simulink model "bicyclemodel22"  (R2015b)
settings: Solver=FixedStepAuto  StartTime=0.0  StopTime=1  FixedStep=0.001  RelTol=1e-3
libraries: simulink x3
settings Model: Creator=ADMIN  LastModifiedBy=ADMIN

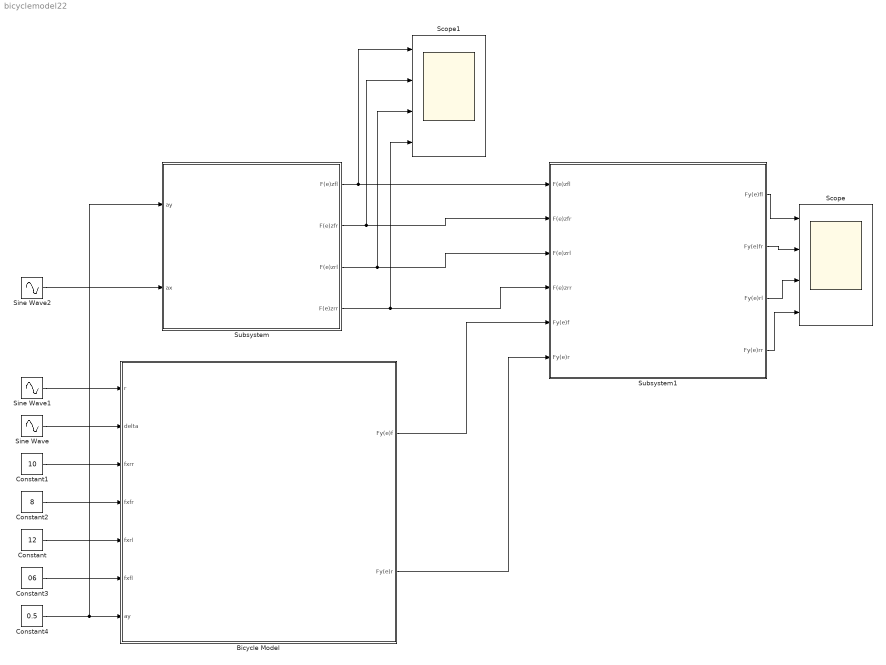
== system bicyclemodel22 ==
  Bicycle Model : Subsystem
  Constant : Constant  Value=12
  Constant1 : Constant  Value=10
  Constant2 : Constant  Value=8
  Constant3 : Constant  Value=06
  Constant4 : Constant  Value=0.5
  Scope : Scope  NumInputPorts=4
  Scope1 : Scope  NumInputPorts=4
  Sine Wave : Sin  Frequency=2
  Sine Wave1 : Sin  Frequency=4
  Sine Wave2 : Sin  Frequency=5
  Subsystem : Subsystem
  Subsystem1 : Subsystem
  wires:
  Subsystem/1(F(e)zfl) -> Scope1/1, Subsystem1/1(F(e)zfl)
  Subsystem/2(F(e)zfr) -> Scope1/2, Subsystem1/2(F(e)zfr)
  Subsystem/3(F(e)zrl) -> Scope1/3, Subsystem1/3(F(e)zrl)
  Subsystem/4(F(e)zrr) -> Scope1/4, Subsystem1/4(F(e)zrr)
  Bicycle Model/1(Fy(e)f) -> Subsystem1/5(Fy(e)f)
  Bicycle Model/2(Fy(e)r) -> Subsystem1/6(Fy(e)r)
  Constant/1 -> Bicycle Model/5(fxrl)
  Sine Wave/1 -> Bicycle Model/2(delta)
  Constant3/1 -> Bicycle Model/6(fxfl)
  Constant2/1 -> Bicycle Model/4(fxfr)
  Constant1/1 -> Bicycle Model/3(fxrr)
  Constant4/1 -> Subsystem/1(ay), Bicycle Model/7(ay)
  Sine Wave1/1 -> Bicycle Model/1(r)
  Subsystem1/1(Fy(e)fl) -> Scope/1
  Sine Wave2/1 -> Subsystem/2(ax)
  Subsystem1/2(Fy(e)fr) -> Scope/2
  Subsystem1/3(Fy(e)rl) -> Scope/3
  Subsystem1/4(Fy(e)rr) -> Scope/4

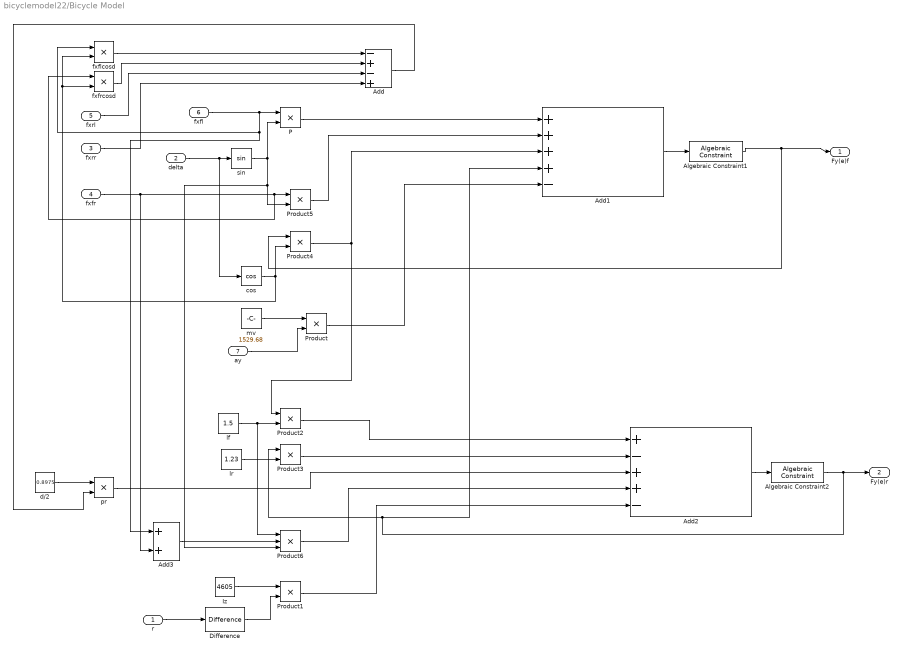
== system bicyclemodel22/Bicycle Model ==
  r : Inport
  delta : Inport  Port=2
  fxrr : Inport  Port=3
  fxfr : Inport  Port=4
  fxrl : Inport  Port=5
  fxfl : Inport  Port=6
  ay : Inport  Port=7
  Add : Sum  Inputs=-+-+
  Add1 : Sum  Inputs=++++-
  Add2 : Sum  Inputs=+-++-
  Add3 : Sum
  Algebraic Constraint1 : simulink/Math Operations/Algebraic Constraint  z0=0
  Algebraic Constraint2 : simulink/Math Operations/Algebraic Constraint  z0=0
  Difference : simulink/Discrete/Difference  ICPrevInput=0.0  InputProcessing=Inherited  OutMin=[]  OutMax=[]  OutDataType=fixdt(1, 16)  OutScaling=2^-10  DoSatur=off
  Iz : Constant  Value=4605
  P : Product
  Product{,1..5} (6 alike) : Product
  Product6 : Product  Inputs=3
  cos : Trigonometry  Operator=cos
  d/2 : Constant  Value=0.8975
  fxflcosd : Product
  fxfrcosd : Product
  lf : Constant  Value=1.5
  lr : Constant  Value=1.23
  mv : Constant  Value=1529.68
  pr : Product
  sin : Trigonometry
  Fy(e)f : Outport
  Fy(e)r : Outport  Port=2
  wires:
  fxfl/1 -> Add3/1, fxflcosd/1, P/1
  fxflcosd/1 -> Add/1
  Add3/1 -> Product6/2
  Add/1 -> pr/2
  Product6/1 -> Add2/4
  fxrr/1 -> Add/4
  fxrl/1 -> Add/3
  Product1/1 -> Add2/5
  fxfrcosd/1 -> Add/2
  r/1 -> Difference/1
  lr/1 -> Product3/2
  lf/1 -> Product6/1, Product2/2
  Product3/1 -> Add2/2
  Product2/1 -> Add2/1
  Iz/1 -> Product1/1
  Algebraic Constraint1/1 -> Product4/1, Fy(e)f/1
  Algebraic Constraint2/1 -> Product3/1, Add1/4, Fy(e)r/1
  mv/1 -> Product/1
  ay/1 -> Product/2
  P/1 -> Add1/1
  delta/1 -> cos/1, sin/1
  Add1/1 -> Algebraic Constraint1/1
  Add2/1 -> Algebraic Constraint2/1
  fxfr/1 -> fxfrcosd/1, Product5/1, Add3/2
  sin/1 -> Product5/2, Product6/3, P/2
  Product5/1 -> Add1/2
  Product4/1 -> Product2/1, Add1/3
  cos/1 -> fxfrcosd/2, fxflcosd/2, Product4/2
  Product/1 -> Add1/5
  d/2/1 -> pr/1
  pr/1 -> Add2/3
  Difference/1 -> Product1/2

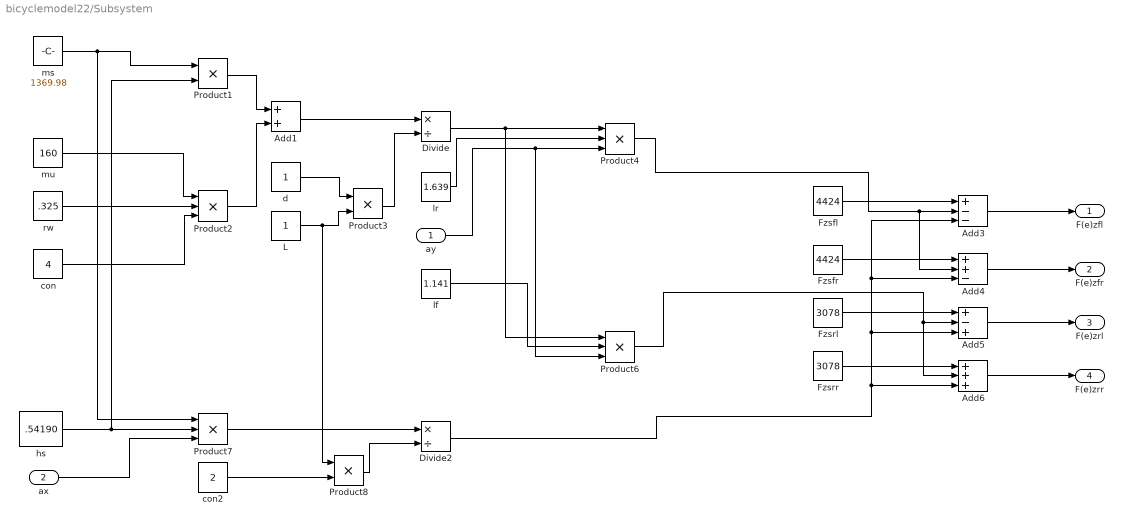
== system bicyclemodel22/Subsystem ==
  ay : Inport
  ax : Inport  Port=2
  Add1 : Sum
  Add3 : Sum  Inputs=+--
  Add4 : Sum  Inputs=++-
  Add5 : Sum  Inputs=+-+
  Add6 : Sum  Inputs=+++
  Divide : Product  Inputs=*/
  Divide2 : Product  Inputs=*/
  Fzsfl : Constant  Value=4424
  Fzsfr : Constant  Value=4424
  Fzsrl : Constant  Value=3078
  Fzsrr : Constant  Value=3078
  L : Constant
  Product1 : Product
  Product{2,4,6..7} (4 alike) : Product  Inputs=3
  Product3 : Product
  Product8 : Product
  con : Constant  Value=4
  con2 : Constant  Value=2
  d : Constant
  hs : Constant  Value=.54190
  lf : Constant  Value=1.141
  lr : Constant  Value=1.639
  ms : Constant  Value=1369.98
  mu : Constant  Value=160
  rw : Constant  Value=.325
  F(e)zfl : Outport
  F(e)zfr : Outport  Port=2
  F(e)zrl : Outport  Port=3
  F(e)zrr : Outport  Port=4
  wires:
  lr/1 -> Product4/2
  ms/1 -> Product7/1, Product1/1
  Divide/1 -> Product6/1, Product4/1
  hs/1 -> Product1/2, Product7/2
  Product3/1 -> Divide/2
  Add1/1 -> Divide/1
  Product1/1 -> Add1/1
  rw/1 -> Product2/2
  Product2/1 -> Add1/2
  mu/1 -> Product2/1
  L/1 -> Product8/1, Product3/2
  d/1 -> Product3/1
  con/1 -> Product2/3
  Product4/1 -> Add4/2, Add3/2
  Product6/1 -> Add6/2, Add5/2
  con2/1 -> Product8/2
  Add6/1 -> F(e)zrr/1
  ax/1 -> Product7/3
  Product7/1 -> Divide2/1
  Fzsrl/1 -> Add5/1
  lf/1 -> Product6/2
  Fzsfl/1 -> Add3/1
  ay/1 -> Product6/3, Product4/3
  Product8/1 -> Divide2/2
  Fzsrr/1 -> Add6/1
  Divide2/1 -> Add6/3, Add5/3, Add4/3, Add3/3
  Add5/1 -> F(e)zrl/1
  Add3/1 -> F(e)zfl/1
  Add4/1 -> F(e)zfr/1
  Fzsfr/1 -> Add4/1

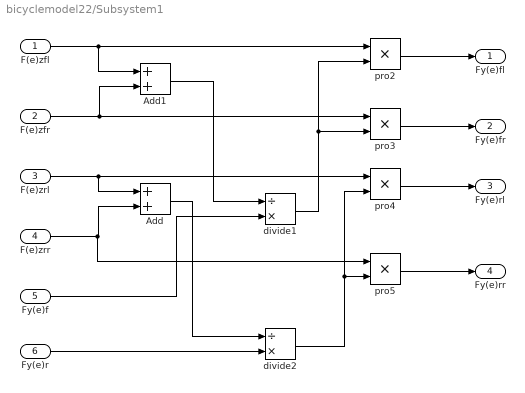
== system bicyclemodel22/Subsystem1 ==
  F(e)zfl : Inport
  F(e)zfr : Inport  Port=2
  F(e)zrl : Inport  Port=3
  F(e)zrr : Inport  Port=4
  Fy(e)f : Inport  Port=5
  Fy(e)r : Inport  Port=6
  Add : Sum
  Add1 : Sum
  divide1 : Product  Inputs=/*
  divide2 : Product  Inputs=/*
  pro{2..5} (4 alike) : Product  Inputs=**
  Fy(e)fl : Outport
  Fy(e)fr : Outport  Port=2
  Fy(e)rl : Outport  Port=3
  Fy(e)rr : Outport  Port=4
  wires:
  Add/1 -> divide2/1
  Fy(e)r/1 -> divide2/2
  F(e)zrl/1 -> pro4/1, Add/1
  divide1/1 -> pro3/2, pro2/2
  pro4/1 -> Fy(e)rl/1
  pro2/1 -> Fy(e)fl/1
  pro3/1 -> Fy(e)fr/1
  Fy(e)f/1 -> divide1/2
  Add1/1 -> divide1/1
  F(e)zfr/1 -> pro3/1, Add1/2
  F(e)zrr/1 -> pro5/1, Add/2
  pro5/1 -> Fy(e)rr/1
  divide2/1 -> pro4/2, pro5/2
  F(e)zfl/1 -> pro2/1, Add1/1
